simulink model "wbs_sim"  (R2025a)
settings: Solver=FixedStepAuto  StartTime=0.0  StopTime=20  FixedStep=0.001  RelTol=1e-3
undefined symbols (not defined in the file or in its folder): dyaw, L_l, L_r, phi_1l, phi_1r, phi_4l, phi_4r, roll, theta_l, theta_r, x, X, Y, yaw, Z
libraries: sm_lib x86, nesl_utility x28, slpidlib x6
(part 1 of 4)
settings Model: Creator=zyh  LastModifiedBy=zyh

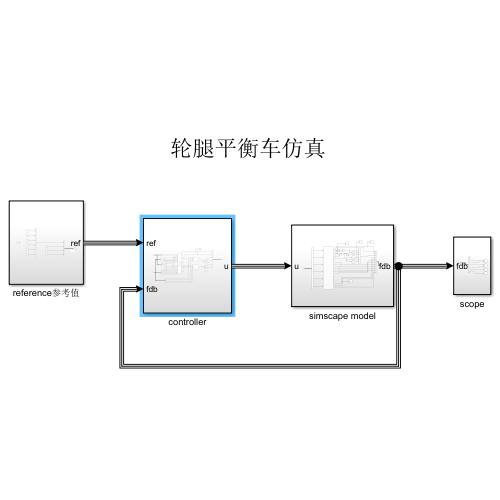
[thumbnail: Simulink's stored preview of the top-level diagram]
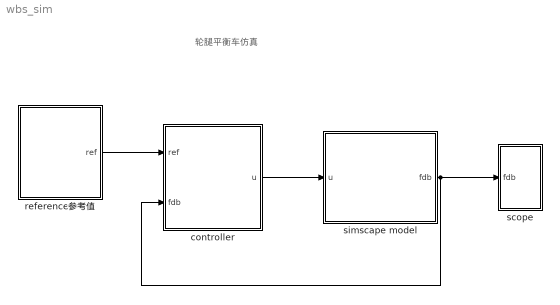
== system wbs_sim ==
  note: 轮腿平衡车仿真
  controller : Subsystem
  reference参考值 : Subsystem
  scope : Subsystem
  simscape model : Subsystem
  wires:
  controller/1(u) -> simscape model/1(u)
  reference参考值/1(ref) -> controller/1(ref)
  simscape model/1(fdb) -> controller/2(fdb), scope/1(fdb)

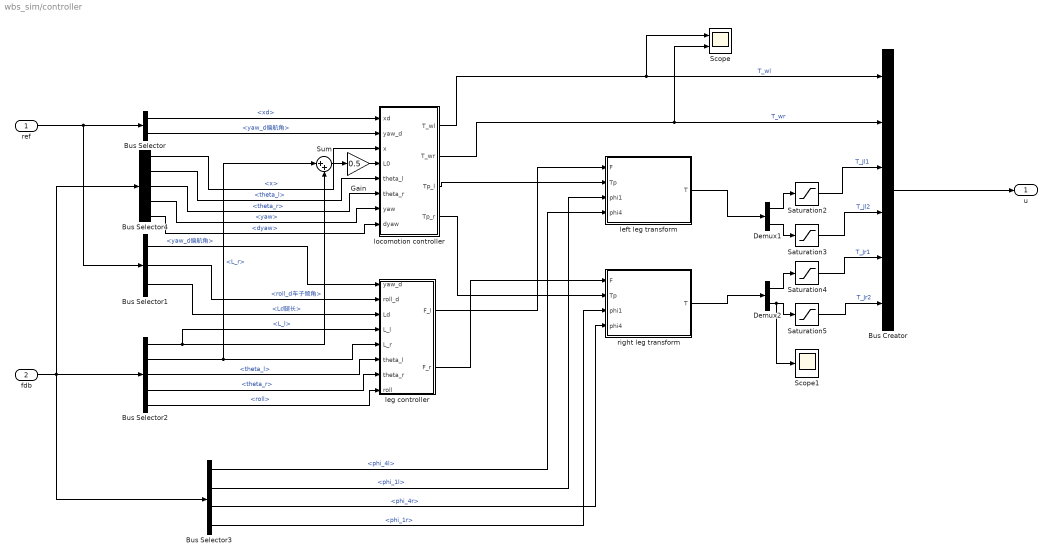
== system wbs_sim/controller ==
  ref : Inport
  fdb : Inport  Port=2
  Bus Creator : BusCreator  Inputs=6
  Bus Selector : BusSelector  OutputSignals=xd,yaw_d偏航角
  Bus Selector1 : BusSelector  OutputSignals=yaw_d偏航角,roll_d车子倾角,Ld腿长
  Bus Selector2 : BusSelector  OutputSignals=L_l,L_r,theta_l,theta_r,roll
  Bus Selector3 : BusSelector  OutputSignals=phi_4l,phi_1l,phi_4r,phi_1r
  Bus Selector4 : BusSelector  OutputSignals=x,theta_l,theta_r,yaw,dyaw
  Demux1 : Demux  Outputs=2
  Demux2 : Demux  Outputs=2
  Gain : Gain  Gain=0.5
  Saturation{2..5} (4 alike) : Saturate  UpperLimit=80  LowerLimit=-80  ZeroCross=off
  Scope : Scope  NumInputPorts=2
      settings: ActiveDisplayYMinimum=-9.67467850137015  ActiveDisplayYMaximum=9.5997754242952382  DataLoggingVariableName=ScopeData6
  Scope1 : Scope
      settings: ActiveDisplayYMinimum=-146.11283015440873  ActiveDisplayYMaximum=330.68518102917665  DataLoggingVariableName=ScopeData13
  Sum : Sum  Inputs=|++
  left leg transform : MATLAB Function  TreatAsAtomicUnit=on
  leg controller : Subsystem
  locomotion controller : Subsystem
  right leg transform : MATLAB Function  TreatAsAtomicUnit=on
  u : Outport
  wires:
  ref/1 -> Bus Selector1/1, Bus Selector/1
  Bus Selector/1 -> locomotion controller/1(xd)  "<xd>"
  Bus Selector/2 -> locomotion controller/2(yaw_d)  "<yaw_d偏航角>"
  Bus Selector1/1 -> leg controller/1(yaw_d)  "<yaw_d偏航角>"
  Bus Selector1/2 -> leg controller/2(roll_d)  "<roll_d车子倾角>"
  Bus Selector1/3 -> leg controller/3(Ld)  "<Ld腿长>"
  Bus Selector2/2 -> leg controller/5(L_r), Sum/1  "<L_r>"
  Bus Selector2/1 -> leg controller/4(L_l), Sum/2  "<L_l>"
  Bus Selector2/4 -> leg controller/7(theta_r)  "<theta_r>"
  Bus Selector2/5 -> leg controller/8(roll)  "<roll>"
  Bus Selector2/3 -> leg controller/6(theta_l)  "<theta_l>"
  Bus Selector4/4 -> locomotion controller/7(yaw)  "<yaw>"
  Bus Selector4/3 -> locomotion controller/6(theta_r)  "<theta_r>"
  Bus Selector4/1 -> locomotion controller/3(x)  "<x>"
  Bus Selector4/2 -> locomotion controller/5(theta_l)  "<theta_l>"
  Bus Selector4/5 -> locomotion controller/8(dyaw)  "<dyaw>"
  fdb/1 -> Bus Selector3/1, Bus Selector4/1, Bus Selector2/1
  Bus Selector3/4 -> right leg transform/3(phi1)  "<phi_1r>"
  Bus Selector3/1 -> left leg transform/4(phi4)  "<phi_4l>"
  Bus Selector3/3 -> right leg transform/4(phi4)  "<phi_4r>"
  Bus Selector3/2 -> left leg transform/3(phi1)  "<phi_1l>"
  Sum/1 -> Gain/1
  Gain/1 -> locomotion controller/4(L0)
  leg controller/1(F_l) -> left leg transform/1(F)
  leg controller/2(F_r) -> right leg transform/1(F)
  locomotion controller/4(Tp_r) -> right leg transform/2(Tp)
  locomotion controller/3(Tp_l) -> left leg transform/2(Tp)
  Bus Creator/1 -> u/1
  left leg transform/1(T) -> Demux1/1
  Saturation4/1 -> Bus Creator/5  "T_Jr1"
  Demux1/1 -> Saturation2/1
  locomotion controller/1(T_wl) -> Scope/1, Bus Creator/1  "T_wl"
  right leg transform/1(T) -> Demux2/1
  Demux2/2 -> Scope1/1, Saturation5/1
  locomotion controller/2(T_wr) -> Scope/2, Bus Creator/2  "T_wr"
  Demux1/2 -> Saturation3/1
  Demux2/1 -> Saturation4/1
  Saturation5/1 -> Bus Creator/6  "T_Jr2"
  Saturation2/1 -> Bus Creator/3  "T_Jl1"
  Saturation3/1 -> Bus Creator/4  "T_Jl2"

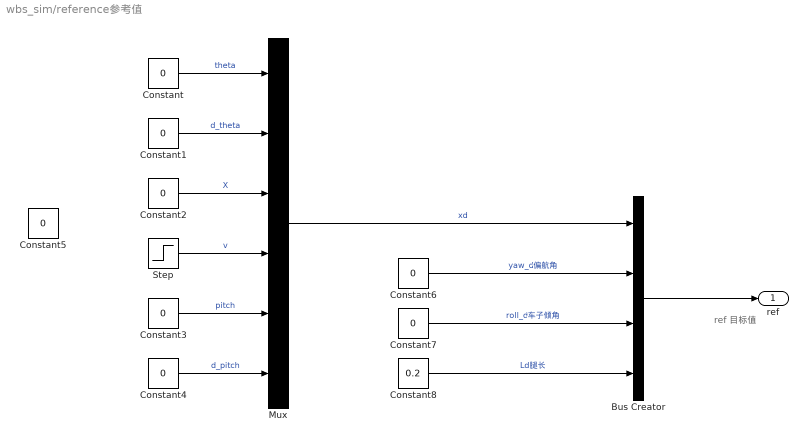
== system wbs_sim/reference参考值 ==
  note: ref
      | 目标值
  Bus Creator : BusCreator  Inputs=4
  Constant{,1..7} (8 alike) : Constant  Value=0
  Constant8 : Constant  Value=0.2
  Mux : Mux  Inputs=6
  Step : Step  Time=3  After=3  SampleTime=0
  ref : Outport
  wires:
  Constant1/1 -> Mux/2  "d_theta"
  Constant2/1 -> Mux/3  "X"
  Constant6/1 -> Bus Creator/2  "yaw_d偏航角"
  Mux/1 -> Bus Creator/1  "xd"
  Constant/1 -> Mux/1  "theta"
  Constant8/1 -> Bus Creator/4  "Ld腿长"
  Bus Creator/1 -> ref/1
  Constant7/1 -> Bus Creator/3  "roll_d车子倾角"
  Constant3/1 -> Mux/5  "pitch"
  Constant4/1 -> Mux/6  "d_pitch"
  Step/1 -> Mux/4  "v"

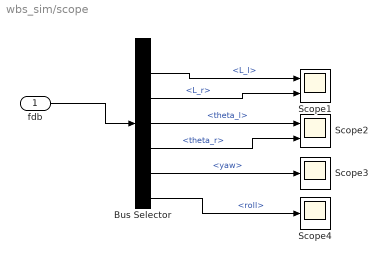
== system wbs_sim/scope ==
  fdb : Inport
  Bus Selector : BusSelector  OutputSignals=x,L_l,L_r,theta_l,theta_r,yaw,roll
  Scope1 : Scope  NumInputPorts=2
      settings: ActiveDisplayYMinimum=0.23913  ActiveDisplayYMaximum=0.25761
  Scope2 : Scope  NumInputPorts=2
      settings: ActiveDisplayYMinimum=-0.29516235436089044  ActiveDisplayYMaximum=0.45341029604825445  DataLoggingVariableName=ScopeData4
  Scope3 : Scope
      settings: ActiveDisplayYMinimum=-0.04188  ActiveDisplayYMaximum=0.02147  DataLoggingVariableName=ScopeData5
  Scope4 : Scope
      settings: ActiveDisplayYMinimum=-0.00154  ActiveDisplayYMaximum=0.00709
  wires:
  fdb/1 -> Bus Selector/1
  Bus Selector/2 -> Scope1/1  "<L_l>"
  Bus Selector/3 -> Scope1/2  "<L_r>"
  Bus Selector/5 -> Scope2/2  "<theta_r>"
  Bus Selector/4 -> Scope2/1  "<theta_l>"
  Bus Selector/6 -> Scope3/1  "<yaw>"
  Bus Selector/7 -> Scope4/1  "<roll>"

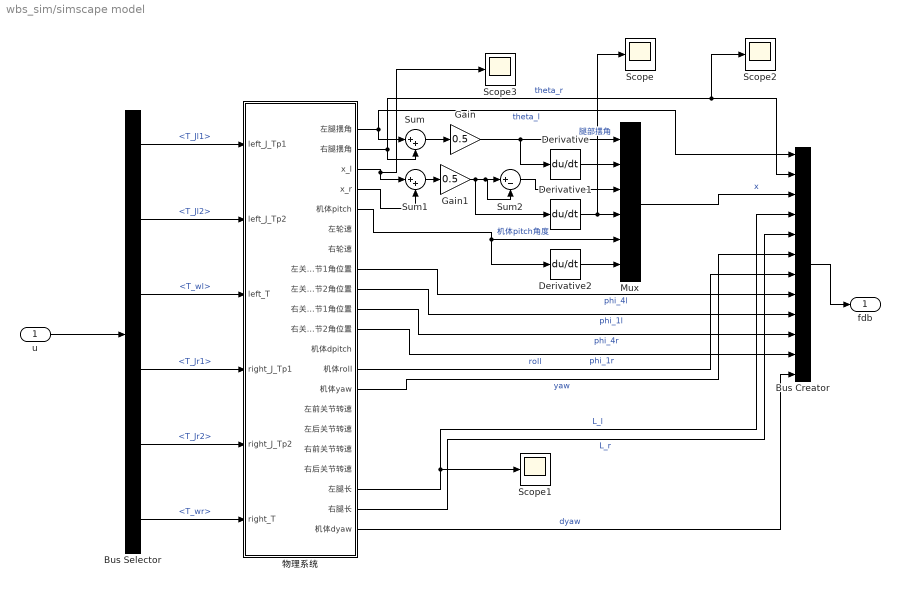
== system wbs_sim/simscape model ==
  u : Inport
  Bus Creator : BusCreator  Inputs=theta_l,theta_r,x,L_l,L_r,yaw,roll,phi_4l,phi_1l,phi_4r,phi_1r,dyaw
  Bus Selector : BusSelector  OutputSignals=T_Jl1,T_Jl2,T_wl,T_Jr1,T_Jr2,T_wr
  Derivative : Derivative
  Derivative1 : Derivative
  Derivative2 : Derivative
  Gain : Gain  Gain=0.5
  Gain1 : Gain  Gain=0.5
  Mux : Mux  Inputs=6
  Scope{,1..3} (4 alike) : Scope
      Scope settings: ActiveDisplayYMinimum=-4.1815375107147821  ActiveDisplayYMaximum=7.1699990036627606  DataLoggingVariableName=ScopeData9
      Scope1 settings: ActiveDisplayYMinimum=-0.014775598665862893  ActiveDisplayYMaximum=0.43261214034743506  DataLoggingVariableName=ScopeData2
      Scope2 settings: ActiveDisplayYMinimum=-0.18066093581675097  ActiveDisplayYMaximum=0.041287187039674843  DataLoggingVariableName=ScopeData15
      Scope3 settings: ActiveDisplayYMinimum=0.91927954446858173  ActiveDisplayYMaximum=1.4817716269099306  DataLoggingVariableName=ScopeData16
  Sum : Sum  Inputs=|++
  Sum1 : Sum  Inputs=|++
  Sum2 : Sum  Inputs=|+-
  物理系统 : Subsystem
  fdb : Outport
  wires:
  u/1 -> Bus Selector/1
  Bus Selector/1 -> 物理系统/1(left_J_Tp1)  "<T_Jl1>"
  Bus Selector/3 -> 物理系统/3(left_T)  "<T_wl>"
  Bus Selector/4 -> 物理系统/4(right_J_Tp1)  "<T_Jr1>"
  Bus Selector/5 -> 物理系统/5(right_J_Tp2)  "<T_Jr2>"
  Bus Selector/6 -> 物理系统/6(right_T)  "<T_wr>"
  Bus Selector/2 -> 物理系统/2(left_J_Tp2)  "<T_Jl2>"
  物理系统/1(左腿摆角) -> Sum/1, Bus Creator/1  "theta_l"
  物理系统/2(右腿摆角) -> Sum/2, Bus Creator/2, Scope2/1  "theta_r"
  Sum/1 -> Gain/1
  Gain/1 -> Derivative/1, Mux/1  "腿部摆角"
  Derivative/1 -> Mux/2
  物理系统/3(x_l) -> Scope3/1, Sum1/1
  物理系统/4(x_r) -> Sum1/2
  Derivative1/1 -> Scope/1, Mux/4
  物理系统/5(机体pitch) -> Mux/5, Derivative2/1  "机体pitch角度"
  Derivative2/1 -> Mux/6
  Mux/1 -> Bus Creator/3  "x"
  Bus Creator/1 -> fdb/1
  物理系统/19(左腿长) -> Bus Creator/4, Scope1/1  "L_l"
  物理系统/20(右腿长) -> Bus Creator/5  "L_r"
  物理系统/14(机体yaw) -> Bus Creator/6  "yaw"
  物理系统/13(机体roll) -> Bus Creator/7  "roll"
  物理系统/8(左关节1角位置) -> Bus Creator/8  "phi_4l"
  物理系统/9(左关节2角位置) -> Bus Creator/9  "phi_1l"
  物理系统/10(右关节1角位置) -> Bus Creator/10  "phi_4r"
  物理系统/11(右关节2角位置) -> Bus Creator/11  "phi_1r"
  物理系统/21(机体dyaw) -> Bus Creator/12  "dyaw"
  Sum1/1 -> Gain1/1
  Gain1/1 -> Derivative1/1, Sum2/2, Sum2/1
  Sum2/1 -> Mux/3

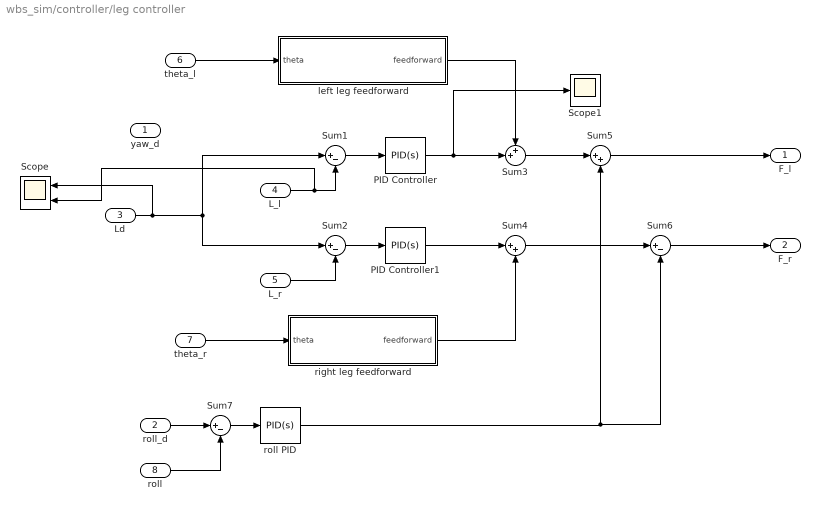
== system wbs_sim/controller/leg controller ==
  yaw_d : Inport
  roll_d : Inport  Port=2
  Ld : Inport  Port=3
  L_l : Inport  Port=4
  L_r : Inport  Port=5
  theta_l : Inport  Port=6
  theta_r : Inport  Port=7
  roll : Inport  Port=8
  PID Controller : slpidlib/PID Controller  Controller=PID  Form=Parallel  TimeDomain=Continuous-time  UseExternalTs=off  SampleTime=-1  IntegratorMethod=Forward Euler  FilterMethod=Forward Euler  ControllerParametersSource=internal  P=4000  I=500  UseKiTs=on  D=500  UseExternalDerivativeSource=off  N=100  UseFilter=on  TunerSelectOption=Transfer Function Based (PID Tuner App)  InitialConditionSource=internal  InitialConditionForIntegrator=0  InitialConditionForFilter=0  DifferentiatorICPrevScaledInput=0  ExternalReset=none  TrackingMode=off  Kt=1  LimitOutput=off  SatLimitsSource=internal  UpperSaturationLimit=1000  LowerSaturationLimit=-1000  LinearizeAsGain=on  AntiWindupMode=none  Kb=1  LimitIntegrator=off  UpperIntegratorSaturationLimit=inf  LowerIntegratorSaturationLimit=-inf  POutMin=[]  POutMax=[]  IOutMin=[]  IOutMax=[]  DOutMin=[]  DOutMax=[]  NOutMin=[]  NOutMax=[]  SumOutMin=[]  SumOutMax=[]  SaturationOutMin=[]  SaturationOutMax=[]  PParamMin=[]  PParamMax=[]  IParamMin=[]  IParamMax=[]  DParamMin=[]  DParamMax=[]  NParamMin=[]  NParamMax=[]  KbParamMin=[]  KbParamMax=[]  KtParamMin=[]  KtParamMax=[]  KbOutMin=[]  KbOutMax=[]  KtOutMin=[]  KtOutMax=[]  IntegratorOutMin=[]  IntegratorOutMax=[]  FilterOutMin=[]  FilterOutMax=[]  SumI1OutMin=[]  SumI1OutMax=[]  SumI2OutMin=[]  SumI2OutMax=[]  SumI3OutMin=[]  SumI3OutMax=[]  SumI4OutMin=[]  SumI4OutMax=[]  SumDOutMin=[]  SumDOutMax=[]  DifferentiatorOutMin=[]  DifferentiatorOutMax=[]  FilterDiffOutCoefMin=[]  FilterDiffOutCoefMax=[]  ReciprocalOutMin=[]  ReciprocalOutMax=[]  SumDenOutMin=[]  SumDenOutMax=[]  SumNumOutMin=[]  SumNumOutMax=[]  DivideOutMin=[]  DivideOutMax=[]  UdiffTsProdOutMin=[]  UdiffTsProdOutMax=[]  NTsProdOutMin=[]  NTsProdOutMax=[]  UintegralTsProdOutMin=[]  UintegralTsProdOutMax=[]  UngainTsProdOutMin=[]  UngainTsProdOutMax=[]  ClampingZeroOutDataTypeStr=Inherit: Inherit via back propagation  ClampingZeroOutMin=[]  ClampingZeroOutMax=[]  FilterDenConstantOutDataTypeStr=Inherit: Inherit via back propagation  FilterDenConstantOutMin=[]  FilterDenConstantOutMax=[]  PCopyOutDataTypeStr=Inherit: Inherit via back propagation  PCopyOutMin=[]  PCopyOutMax=[]  NCopyOutDataTypeStr=Inherit: Inherit via back propagation  NCopyOutMin=[]  NCopyOutMax=[]  IntegratorContinuousStateAttributes=''  IntegratorStateMustResolveToSignalObject=off  IntegratorRTWStateStorageClass=Auto  FilterContinuousStateAttributes=''  FilterStateMustResolveToSignalObject=off  FilterRTWStateStorageClass=Auto  ParallelPVariant=InternalParameters  IdealPVariant=Disabled  IVariant=InternalParameters  DVariant=InternalParameters  IntegratorVariant=Continuous  SatVariant=Disabled  AWVariant=Passthrough  PCopyVariant=Disabled  TRVariant=Disabled  FdbkBlocksVariant=Forward  IdealPFdbkVariant=Disabled  SatFdbkVariant=Disabled  DerivativeFilterVariant=ContFilter  NVariant=InternalParameters  NCopyVariant=Disabled  FilterICVariant=InternalICsFilter  IntegratorICVariant=InternalICs  ExternalResetVariant=Disabled  TRSumVariant=Passthrough  SumFdbkVariant=Disabled  SumVariant=Sum_PID  TsampFilterVariant=InternalTs  TsampNgainVariant=Passthrough  TsampIntegralVariant=Disabled_SignalSpec  ExternalSaturationOutDataTypeStr=Inherit: Same as second input  DerivativeSourceVariant=ErrorSignal  PreIntVariant=InternalPreInt
  PID Controller1 : slpidlib/PID Controller  Controller=PID  Form=Parallel  TimeDomain=Continuous-time  UseExternalTs=off  SampleTime=-1  IntegratorMethod=Forward Euler  FilterMethod=Forward Euler  ControllerParametersSource=internal  P=4000  I=500  UseKiTs=on  D=500  UseExternalDerivativeSource=off  N=100  UseFilter=on  TunerSelectOption=Transfer Function Based (PID Tuner App)  InitialConditionSource=internal  InitialConditionForIntegrator=0  InitialConditionForFilter=0  DifferentiatorICPrevScaledInput=0  ExternalReset=none  TrackingMode=off  Kt=1  LimitOutput=off  SatLimitsSource=internal  UpperSaturationLimit=1000  LowerSaturationLimit=-1000  LinearizeAsGain=on  AntiWindupMode=none  Kb=1  LimitIntegrator=off  UpperIntegratorSaturationLimit=inf  LowerIntegratorSaturationLimit=-inf  POutMin=[]  POutMax=[]  IOutMin=[]  IOutMax=[]  DOutMin=[]  DOutMax=[]  NOutMin=[]  NOutMax=[]  SumOutMin=[]  SumOutMax=[]  SaturationOutMin=[]  SaturationOutMax=[]  PParamMin=[]  PParamMax=[]  IParamMin=[]  IParamMax=[]  DParamMin=[]  DParamMax=[]  NParamMin=[]  NParamMax=[]  KbParamMin=[]  KbParamMax=[]  KtParamMin=[]  KtParamMax=[]  KbOutMin=[]  KbOutMax=[]  KtOutMin=[]  KtOutMax=[]  IntegratorOutMin=[]  IntegratorOutMax=[]  FilterOutMin=[]  FilterOutMax=[]  SumI1OutMin=[]  SumI1OutMax=[]  SumI2OutMin=[]  SumI2OutMax=[]  SumI3OutMin=[]  SumI3OutMax=[]  SumI4OutMin=[]  SumI4OutMax=[]  SumDOutMin=[]  SumDOutMax=[]  DifferentiatorOutMin=[]  DifferentiatorOutMax=[]  FilterDiffOutCoefMin=[]  FilterDiffOutCoefMax=[]  ReciprocalOutMin=[]  ReciprocalOutMax=[]  SumDenOutMin=[]  SumDenOutMax=[]  SumNumOutMin=[]  SumNumOutMax=[]  DivideOutMin=[]  DivideOutMax=[]  UdiffTsProdOutMin=[]  UdiffTsProdOutMax=[]  NTsProdOutMin=[]  NTsProdOutMax=[]  UintegralTsProdOutMin=[]  UintegralTsProdOutMax=[]  UngainTsProdOutMin=[]  UngainTsProdOutMax=[]  ClampingZeroOutDataTypeStr=Inherit: Inherit via back propagation  ClampingZeroOutMin=[]  ClampingZeroOutMax=[]  FilterDenConstantOutDataTypeStr=Inherit: Inherit via back propagation  FilterDenConstantOutMin=[]  FilterDenConstantOutMax=[]  PCopyOutDataTypeStr=Inherit: Inherit via back propagation  PCopyOutMin=[]  PCopyOutMax=[]  NCopyOutDataTypeStr=Inherit: Inherit via back propagation  NCopyOutMin=[]  NCopyOutMax=[]  IntegratorContinuousStateAttributes=''  IntegratorStateMustResolveToSignalObject=off  IntegratorRTWStateStorageClass=Auto  FilterContinuousStateAttributes=''  FilterStateMustResolveToSignalObject=off  FilterRTWStateStorageClass=Auto  ParallelPVariant=InternalParameters  IdealPVariant=Disabled  IVariant=InternalParameters  DVariant=InternalParameters  IntegratorVariant=Continuous  SatVariant=Disabled  AWVariant=Passthrough  PCopyVariant=Disabled  TRVariant=Disabled  FdbkBlocksVariant=Forward  IdealPFdbkVariant=Disabled  SatFdbkVariant=Disabled  DerivativeFilterVariant=ContFilter  NVariant=InternalParameters  NCopyVariant=Disabled  FilterICVariant=InternalICsFilter  IntegratorICVariant=InternalICs  ExternalResetVariant=Disabled  TRSumVariant=Passthrough  SumFdbkVariant=Disabled  SumVariant=Sum_PID  TsampFilterVariant=InternalTs  TsampNgainVariant=Passthrough  TsampIntegralVariant=Disabled_SignalSpec  ExternalSaturationOutDataTypeStr=Inherit: Same as second input  DerivativeSourceVariant=ErrorSignal  PreIntVariant=InternalPreInt
  Scope : Scope  NumInputPorts=2
      settings: ActiveDisplayYMinimum=0.12956670112277244  ActiveDisplayYMaximum=0.27689382263080864  DataLoggingVariableName=ScopeData11
  Scope1 : Scope
      settings: ActiveDisplayYMinimum=-63.72645961170668  ActiveDisplayYMaximum=-21.722148449495378  DataLoggingVariableName=ScopeData12
  Sum{1..2,6..7} (4 alike) : Sum  Inputs=|+-
  Sum3 : Sum  Inputs=++|
  Sum4 : Sum  Inputs=|++
  Sum5 : Sum  Inputs=|++
  left leg feedforward : MATLAB Function  TreatAsAtomicUnit=on
  right leg feedforward : MATLAB Function  TreatAsAtomicUnit=on
  roll PID : slpidlib/PID Controller  Controller=PID  Form=Parallel  TimeDomain=Continuous-time  UseExternalTs=off  SampleTime=-1  IntegratorMethod=Forward Euler  FilterMethod=Forward Euler  ControllerParametersSource=internal  P=500  I=500  UseKiTs=off  D=200  UseExternalDerivativeSource=off  N=100  UseFilter=on  TunerSelectOption=Transfer Function Based (PID Tuner App)  InitialConditionSource=internal  InitialConditionForIntegrator=0  InitialConditionForFilter=0  DifferentiatorICPrevScaledInput=0  ExternalReset=none  TrackingMode=off  Kt=1  LimitOutput=off  SatLimitsSource=internal  UpperSaturationLimit=inf  LowerSaturationLimit=-inf  LinearizeAsGain=on  AntiWindupMode=none  Kb=1  LimitIntegrator=off  UpperIntegratorSaturationLimit=1.5  LowerIntegratorSaturationLimit=-1.5  POutMin=[]  POutMax=[]  IOutMin=[]  IOutMax=[]  DOutMin=[]  DOutMax=[]  NOutMin=[]  NOutMax=[]  SumOutMin=[]  SumOutMax=[]  SaturationOutMin=[]  SaturationOutMax=[]  PParamMin=[]  PParamMax=[]  IParamMin=[]  IParamMax=[]  DParamMin=[]  DParamMax=[]  NParamMin=[]  NParamMax=[]  KbParamMin=[]  KbParamMax=[]  KtParamMin=[]  KtParamMax=[]  KbOutMin=[]  KbOutMax=[]  KtOutMin=[]  KtOutMax=[]  IntegratorOutMin=[]  IntegratorOutMax=[]  FilterOutMin=[]  FilterOutMax=[]  SumI1OutMin=[]  SumI1OutMax=[]  SumI2OutMin=[]  SumI2OutMax=[]  SumI3OutMin=[]  SumI3OutMax=[]  SumI4OutMin=[]  SumI4OutMax=[]  SumDOutMin=[]  SumDOutMax=[]  DifferentiatorOutMin=[]  DifferentiatorOutMax=[]  FilterDiffOutCoefMin=[]  FilterDiffOutCoefMax=[]  ReciprocalOutMin=[]  ReciprocalOutMax=[]  SumDenOutMin=[]  SumDenOutMax=[]  SumNumOutMin=[]  SumNumOutMax=[]  DivideOutMin=[]  DivideOutMax=[]  UdiffTsProdOutMin=[]  UdiffTsProdOutMax=[]  NTsProdOutMin=[]  NTsProdOutMax=[]  UintegralTsProdOutMin=[]  UintegralTsProdOutMax=[]  UngainTsProdOutMin=[]  UngainTsProdOutMax=[]  ClampingZeroOutDataTypeStr=Inherit: Inherit via back propagation  ClampingZeroOutMin=[]  ClampingZeroOutMax=[]  FilterDenConstantOutDataTypeStr=Inherit: Inherit via back propagation  FilterDenConstantOutMin=[]  FilterDenConstantOutMax=[]  PCopyOutDataTypeStr=Inherit: Inherit via back propagation  PCopyOutMin=[]  PCopyOutMax=[]  NCopyOutDataTypeStr=Inherit: Inherit via back propagation  NCopyOutMin=[]  NCopyOutMax=[]  IntegratorContinuousStateAttributes=''  IntegratorStateMustResolveToSignalObject=off  IntegratorRTWStateStorageClass=Auto  FilterContinuousStateAttributes=''  FilterStateMustResolveToSignalObject=off  FilterRTWStateStorageClass=Auto  ParallelPVariant=InternalParameters  IdealPVariant=Disabled  IVariant=InternalParameters  DVariant=InternalParameters  IntegratorVariant=Continuous  SatVariant=Disabled  AWVariant=Passthrough  PCopyVariant=Disabled  TRVariant=Disabled  FdbkBlocksVariant=Forward  IdealPFdbkVariant=Disabled  SatFdbkVariant=Disabled  DerivativeFilterVariant=ContFilter  NVariant=InternalParameters  NCopyVariant=Disabled  FilterICVariant=InternalICsFilter  IntegratorICVariant=InternalICs  ExternalResetVariant=Disabled  TRSumVariant=Passthrough  SumFdbkVariant=Disabled  SumVariant=Sum_PID  TsampFilterVariant=InternalTs  TsampNgainVariant=Passthrough  TsampIntegralVariant=Disabled_SignalSpec  ExternalSaturationOutDataTypeStr=Inherit: Same as second input  DerivativeSourceVariant=ErrorSignal  PreIntVariant=InternalPreInt
  F_l : Outport
  F_r : Outport  Port=2
  wires:
  roll_d/1 -> Sum7/1
  L_l/1 -> Scope/2, Sum1/2
  roll/1 -> Sum7/2
  PID Controller1/1 -> Sum4/1
  Sum5/1 -> F_l/1
  theta_r/1 -> right leg feedforward/1(theta)
  theta_l/1 -> left leg feedforward/1(theta)
  Sum1/1 -> PID Controller/1
  L_r/1 -> Sum2/2
  Sum3/1 -> Sum5/1
  PID Controller/1 -> Scope1/1, Sum3/2
  Sum4/1 -> Sum6/1
  Sum6/1 -> F_r/1
  Sum7/1 -> roll PID/1
  roll PID/1 -> Sum6/2, Sum5/2
  left leg feedforward/1(feedforward) -> Sum3/1
  Sum2/1 -> PID Controller1/1
  right leg feedforward/1(feedforward) -> Sum4/2
  Ld/1 -> Scope/1, Sum1/1, Sum2/1

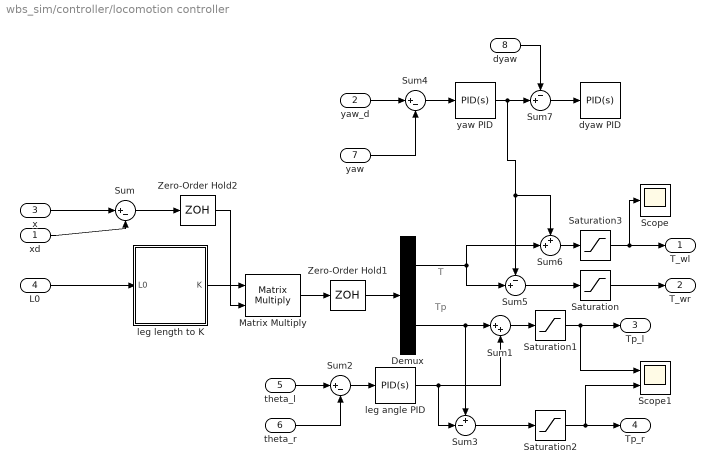
== system wbs_sim/controller/locomotion controller ==
  note: Tp
  note: T
  xd : Inport
  yaw_d : Inport  Port=2
  x : Inport  Port=3
  L0 : Inport  Port=4
  theta_l : Inport  Port=5
  theta_r : Inport  Port=6
  yaw : Inport  Port=7
  dyaw : Inport  Port=8
  Demux : Demux  Outputs=2
  Matrix Multiply : Product  Multiplication=Matrix(*)
  Saturation : Saturate  UpperLimit=4  LowerLimit=-4  ZeroCross=off
  Saturation1 : Saturate  UpperLimit=50  LowerLimit=-50  ZeroCross=off
  Saturation2 : Saturate  UpperLimit=50  LowerLimit=-50  ZeroCross=off
  Saturation3 : Saturate  UpperLimit=4  LowerLimit=-4  ZeroCross=off
  Scope : Scope
      settings: ActiveDisplayYMinimum=-20.083677255725213  ActiveDisplayYMaximum=15.473049623718445  DataLoggingVariableName=ScopeData3
  Scope1 : Scope  NumInputPorts=2
      settings: ActiveDisplayYMinimum=-21.2962391598946  ActiveDisplayYMaximum=19.400174064703325  DataLoggingVariableName=ScopeData14
  Sum : Sum  Inputs=|+-
  Sum1 : Sum  Inputs=|++
  Sum2 : Sum  Inputs=|+-
  Sum3 : Sum  Inputs=+-|
  Sum4 : Sum  Inputs=|+-
  Sum5 : Sum  Inputs=-+|
  Sum6 : Sum  Inputs=++|
  Sum7 : Sum  Inputs=-+|
  Zero-Order Hold1 : ZeroOrderHold  SampleTime=0.001
  Zero-Order Hold2 : ZeroOrderHold  SampleTime=0.001
  dyaw PID : slpidlib/PID Controller  Controller=PID  Form=Parallel  TimeDomain=Continuous-time  UseExternalTs=off  SampleTime=-1  IntegratorMethod=Forward Euler  FilterMethod=Forward Euler  ControllerParametersSource=internal  P=1  I=0.1  UseKiTs=off  D=1  UseExternalDerivativeSource=off  N=100  UseFilter=on  TunerSelectOption=Transfer Function Based (PID Tuner App)  InitialConditionSource=internal  InitialConditionForIntegrator=0  InitialConditionForFilter=0  DifferentiatorICPrevScaledInput=0  ExternalReset=none  TrackingMode=off  Kt=1  LimitOutput=off  SatLimitsSource=internal  UpperSaturationLimit=inf  LowerSaturationLimit=-inf  LinearizeAsGain=on  AntiWindupMode=none  Kb=1  LimitIntegrator=off  UpperIntegratorSaturationLimit=1.5  LowerIntegratorSaturationLimit=-1.5  POutMin=[]  POutMax=[]  IOutMin=[]  IOutMax=[]  DOutMin=[]  DOutMax=[]  NOutMin=[]  NOutMax=[]  SumOutMin=[]  SumOutMax=[]  SaturationOutMin=[]  SaturationOutMax=[]  PParamMin=[]  PParamMax=[]  IParamMin=[]  IParamMax=[]  DParamMin=[]  DParamMax=[]  NParamMin=[]  NParamMax=[]  KbParamMin=[]  KbParamMax=[]  KtParamMin=[]  KtParamMax=[]  KbOutMin=[]  KbOutMax=[]  KtOutMin=[]  KtOutMax=[]  IntegratorOutMin=[]  IntegratorOutMax=[]  FilterOutMin=[]  FilterOutMax=[]  SumI1OutMin=[]  SumI1OutMax=[]  SumI2OutMin=[]  SumI2OutMax=[]  SumI3OutMin=[]  SumI3OutMax=[]  SumI4OutMin=[]  SumI4OutMax=[]  SumDOutMin=[]  SumDOutMax=[]  DifferentiatorOutMin=[]  DifferentiatorOutMax=[]  FilterDiffOutCoefMin=[]  FilterDiffOutCoefMax=[]  ReciprocalOutMin=[]  ReciprocalOutMax=[]  SumDenOutMin=[]  SumDenOutMax=[]  SumNumOutMin=[]  SumNumOutMax=[]  DivideOutMin=[]  DivideOutMax=[]  UdiffTsProdOutMin=[]  UdiffTsProdOutMax=[]  NTsProdOutMin=[]  NTsProdOutMax=[]  UintegralTsProdOutMin=[]  UintegralTsProdOutMax=[]  UngainTsProdOutMin=[]  UngainTsProdOutMax=[]  ClampingZeroOutDataTypeStr=Inherit: Inherit via back propagation  ClampingZeroOutMin=[]  ClampingZeroOutMax=[]  FilterDenConstantOutDataTypeStr=Inherit: Inherit via back propagation  FilterDenConstantOutMin=[]  FilterDenConstantOutMax=[]  PCopyOutDataTypeStr=Inherit: Inherit via back propagation  PCopyOutMin=[]  PCopyOutMax=[]  NCopyOutDataTypeStr=Inherit: Inherit via back propagation  NCopyOutMin=[]  NCopyOutMax=[]  IntegratorContinuousStateAttributes=''  IntegratorStateMustResolveToSignalObject=off  IntegratorRTWStateStorageClass=Auto  FilterContinuousStateAttributes=''  FilterStateMustResolveToSignalObject=off  FilterRTWStateStorageClass=Auto  ParallelPVariant=InternalParameters  IdealPVariant=Disabled  IVariant=InternalParameters  DVariant=InternalParameters  IntegratorVariant=Continuous  SatVariant=Disabled  AWVariant=Passthrough  PCopyVariant=Disabled  TRVariant=Disabled  FdbkBlocksVariant=Forward  IdealPFdbkVariant=Disabled  SatFdbkVariant=Disabled  DerivativeFilterVariant=ContFilter  NVariant=InternalParameters  NCopyVariant=Disabled  FilterICVariant=InternalICsFilter  IntegratorICVariant=InternalICs  ExternalResetVariant=Disabled  TRSumVariant=Passthrough  SumFdbkVariant=Disabled  SumVariant=Sum_PID  TsampFilterVariant=InternalTs  TsampNgainVariant=Passthrough  TsampIntegralVariant=Disabled_SignalSpec  ExternalSaturationOutDataTypeStr=Inherit: Same as second input  DerivativeSourceVariant=ErrorSignal  PreIntVariant=InternalPreInt
  leg angle PID : slpidlib/PID Controller  Controller=PID  Form=Parallel  TimeDomain=Continuous-time  UseExternalTs=off  SampleTime=-1  IntegratorMethod=Forward Euler  FilterMethod=Forward Euler  ControllerParametersSource=internal  P=500  I=200  UseKiTs=off  D=200  UseExternalDerivativeSource=off  N=100  UseFilter=on  TunerSelectOption=Transfer Function Based (PID Tuner App)  InitialConditionSource=internal  InitialConditionForIntegrator=0  InitialConditionForFilter=0  DifferentiatorICPrevScaledInput=0  ExternalReset=none  TrackingMode=off  Kt=1  LimitOutput=off  SatLimitsSource=internal  UpperSaturationLimit=inf  LowerSaturationLimit=-inf  LinearizeAsGain=on  AntiWindupMode=none  Kb=1  LimitIntegrator=off  UpperIntegratorSaturationLimit=1.5  LowerIntegratorSaturationLimit=-1.5  POutMin=[]  POutMax=[]  IOutMin=[]  IOutMax=[]  DOutMin=[]  DOutMax=[]  NOutMin=[]  NOutMax=[]  SumOutMin=[]  SumOutMax=[]  SaturationOutMin=[]  SaturationOutMax=[]  PParamMin=[]  PParamMax=[]  IParamMin=[]  IParamMax=[]  DParamMin=[]  DParamMax=[]  NParamMin=[]  NParamMax=[]  KbParamMin=[]  KbParamMax=[]  KtParamMin=[]  KtParamMax=[]  KbOutMin=[]  KbOutMax=[]  KtOutMin=[]  KtOutMax=[]  IntegratorOutMin=[]  IntegratorOutMax=[]  FilterOutMin=[]  FilterOutMax=[]  SumI1OutMin=[]  SumI1OutMax=[]  SumI2OutMin=[]  SumI2OutMax=[]  SumI3OutMin=[]  SumI3OutMax=[]  SumI4OutMin=[]  SumI4OutMax=[]  SumDOutMin=[]  SumDOutMax=[]  DifferentiatorOutMin=[]  DifferentiatorOutMax=[]  FilterDiffOutCoefMin=[]  FilterDiffOutCoefMax=[]  ReciprocalOutMin=[]  ReciprocalOutMax=[]  SumDenOutMin=[]  SumDenOutMax=[]  SumNumOutMin=[]  SumNumOutMax=[]  DivideOutMin=[]  DivideOutMax=[]  UdiffTsProdOutMin=[]  UdiffTsProdOutMax=[]  NTsProdOutMin=[]  NTsProdOutMax=[]  UintegralTsProdOutMin=[]  UintegralTsProdOutMax=[]  UngainTsProdOutMin=[]  UngainTsProdOutMax=[]  ClampingZeroOutDataTypeStr=Inherit: Inherit via back propagation  ClampingZeroOutMin=[]  ClampingZeroOutMax=[]  FilterDenConstantOutDataTypeStr=Inherit: Inherit via back propagation  FilterDenConstantOutMin=[]  FilterDenConstantOutMax=[]  PCopyOutDataTypeStr=Inherit: Inherit via back propagation  PCopyOutMin=[]  PCopyOutMax=[]  NCopyOutDataTypeStr=Inherit: Inherit via back propagation  NCopyOutMin=[]  NCopyOutMax=[]  IntegratorContinuousStateAttributes=''  IntegratorStateMustResolveToSignalObject=off  IntegratorRTWStateStorageClass=Auto  FilterContinuousStateAttributes=''  FilterStateMustResolveToSignalObject=off  FilterRTWStateStorageClass=Auto  ParallelPVariant=InternalParameters  IdealPVariant=Disabled  IVariant=InternalParameters  DVariant=InternalParameters  IntegratorVariant=Continuous  SatVariant=Disabled  AWVariant=Passthrough  PCopyVariant=Disabled  TRVariant=Disabled  FdbkBlocksVariant=Forward  IdealPFdbkVariant=Disabled  SatFdbkVariant=Disabled  DerivativeFilterVariant=ContFilter  NVariant=InternalParameters  NCopyVariant=Disabled  FilterICVariant=InternalICsFilter  IntegratorICVariant=InternalICs  ExternalResetVariant=Disabled  TRSumVariant=Passthrough  SumFdbkVariant=Disabled  SumVariant=Sum_PID  TsampFilterVariant=InternalTs  TsampNgainVariant=Passthrough  TsampIntegralVariant=Disabled_SignalSpec  ExternalSaturationOutDataTypeStr=Inherit: Same as second input  DerivativeSourceVariant=ErrorSignal  PreIntVariant=InternalPreInt
  leg length to K : MATLAB Function  TreatAsAtomicUnit=on
  yaw PID : slpidlib/PID Controller  Controller=PID  Form=Parallel  TimeDomain=Continuous-time  UseExternalTs=off  SampleTime=-1  IntegratorMethod=Forward Euler  FilterMethod=Forward Euler  ControllerParametersSource=internal  P=2  I=0.3  UseKiTs=off  D=2  UseExternalDerivativeSource=off  N=100  UseFilter=on  TunerSelectOption=Transfer Function Based (PID Tuner App)  InitialConditionSource=internal  InitialConditionForIntegrator=0  InitialConditionForFilter=0  DifferentiatorICPrevScaledInput=0  ExternalReset=none  TrackingMode=off  Kt=1  LimitOutput=off  SatLimitsSource=internal  UpperSaturationLimit=inf  LowerSaturationLimit=-inf  LinearizeAsGain=on  AntiWindupMode=none  Kb=1  LimitIntegrator=off  UpperIntegratorSaturationLimit=1.5  LowerIntegratorSaturationLimit=-1.5  POutMin=[]  POutMax=[]  IOutMin=[]  IOutMax=[]  DOutMin=[]  DOutMax=[]  NOutMin=[]  NOutMax=[]  SumOutMin=[]  SumOutMax=[]  SaturationOutMin=[]  SaturationOutMax=[]  PParamMin=[]  PParamMax=[]  IParamMin=[]  IParamMax=[]  DParamMin=[]  DParamMax=[]  NParamMin=[]  NParamMax=[]  KbParamMin=[]  KbParamMax=[]  KtParamMin=[]  KtParamMax=[]  KbOutMin=[]  KbOutMax=[]  KtOutMin=[]  KtOutMax=[]  IntegratorOutMin=[]  IntegratorOutMax=[]  FilterOutMin=[]  FilterOutMax=[]  SumI1OutMin=[]  SumI1OutMax=[]  SumI2OutMin=[]  SumI2OutMax=[]  SumI3OutMin=[]  SumI3OutMax=[]  SumI4OutMin=[]  SumI4OutMax=[]  SumDOutMin=[]  SumDOutMax=[]  DifferentiatorOutMin=[]  DifferentiatorOutMax=[]  FilterDiffOutCoefMin=[]  FilterDiffOutCoefMax=[]  ReciprocalOutMin=[]  ReciprocalOutMax=[]  SumDenOutMin=[]  SumDenOutMax=[]  SumNumOutMin=[]  SumNumOutMax=[]  DivideOutMin=[]  DivideOutMax=[]  UdiffTsProdOutMin=[]  UdiffTsProdOutMax=[]  NTsProdOutMin=[]  NTsProdOutMax=[]  UintegralTsProdOutMin=[]  UintegralTsProdOutMax=[]  UngainTsProdOutMin=[]  UngainTsProdOutMax=[]  ClampingZeroOutDataTypeStr=Inherit: Inherit via back propagation  ClampingZeroOutMin=[]  ClampingZeroOutMax=[]  FilterDenConstantOutDataTypeStr=Inherit: Inherit via back propagation  FilterDenConstantOutMin=[]  FilterDenConstantOutMax=[]  PCopyOutDataTypeStr=Inherit: Inherit via back propagation  PCopyOutMin=[]  PCopyOutMax=[]  NCopyOutDataTypeStr=Inherit: Inherit via back propagation  NCopyOutMin=[]  NCopyOutMax=[]  IntegratorContinuousStateAttributes=''  IntegratorStateMustResolveToSignalObject=off  IntegratorRTWStateStorageClass=Auto  FilterContinuousStateAttributes=''  FilterStateMustResolveToSignalObject=off  FilterRTWStateStorageClass=Auto  ParallelPVariant=InternalParameters  IdealPVariant=Disabled  IVariant=InternalParameters  DVariant=InternalParameters  IntegratorVariant=Continuous  SatVariant=Disabled  AWVariant=Passthrough  PCopyVariant=Disabled  TRVariant=Disabled  FdbkBlocksVariant=Forward  IdealPFdbkVariant=Disabled  SatFdbkVariant=Disabled  DerivativeFilterVariant=ContFilter  NVariant=InternalParameters  NCopyVariant=Disabled  FilterICVariant=InternalICsFilter  IntegratorICVariant=InternalICs  ExternalResetVariant=Disabled  TRSumVariant=Passthrough  SumFdbkVariant=Disabled  SumVariant=Sum_PID  TsampFilterVariant=InternalTs  TsampNgainVariant=Passthrough  TsampIntegralVariant=Disabled_SignalSpec  ExternalSaturationOutDataTypeStr=Inherit: Same as second input  DerivativeSourceVariant=ErrorSignal  PreIntVariant=InternalPreInt
  T_wl : Outport
  T_wr : Outport  Port=2
  Tp_l : Outport  Port=3
  Tp_r : Outport  Port=4
  wires:
  Sum4/1 -> yaw PID/1
  Demux/2 -> Sum1/1, Sum3/1
  Sum3/1 -> Saturation2/1
  yaw PID/1 -> Sum7/2, Sum6/1, Sum5/1
  Saturation1/1 -> Scope1/1, Tp_l/1
  yaw/1 -> Sum4/2
  Sum6/1 -> Saturation3/1
  Sum2/1 -> leg angle PID/1
  Sum1/1 -> Saturation1/1
  Zero-Order Hold1/1 -> Demux/1
  Saturation2/1 -> Scope1/2, Tp_r/1
  Sum5/1 -> Saturation/1
  Demux/1 -> Sum6/2, Sum5/2
  dyaw/1 -> Sum7/1
  Sum7/1 -> dyaw PID/1
  theta_l/1 -> Sum2/1
  x/1 -> Sum/1
  yaw_d/1 -> Sum4/1
  L0/1 -> leg length to K/1(L0)
  Zero-Order Hold2/1 -> Matrix Multiply/2
  Saturation/1 -> T_wr/1
  Saturation3/1 -> Scope/1, T_wl/1
  Matrix Multiply/1 -> Zero-Order Hold1/1
  leg angle PID/1 -> Sum1/2, Sum3/2
  leg length to K/1(K) -> Matrix Multiply/1
  Sum/1 -> Zero-Order Hold2/1
  theta_r/1 -> Sum2/2
  xd/1 -> Sum/2
